simulink model "TorqueCtrl"  (R2022b)
settings: Solver=FixedStepDiscrete  StartTime=0.0  StopTime=10.0  RelTol=1e-3
values from neighbouring files (symbols this model uses):
  C_TorqueCtrl_MaxTrqIndex_u16 = 0.0    [TorqueCtrl.sldd]    (also in TorqueCtrl_objects.m = myPackage.Parameter)
  C_TorqueCtrl_MaxTrqTable_u16 = 0.0    [TorqueCtrl.sldd]    (also in TorqueCtrl_objects.m = myPackage.Parameter)
  C_TorqueCtrl_PowerCoeff60V_u16 = 0.0    [TorqueCtrl.sldd]    (also in TorqueCtrl_objects.m = myPackage.Parameter)
  C_TorqueCtrl_PowerCoeff72V_u16 = 0.0    [TorqueCtrl.sldd]    (also in TorqueCtrl_objects.m = myPackage.Parameter)
undefined symbols (not defined in the file or in its folder): ANALOG, cSpeedLoopMode, cTorqueLoopMode, MOTORDIR, ParamCfg_CommandSource_u16, ParamCfg_MaxSpeed_u16, ParamCfg_PowerMax_u16, ParamCfg_PowerMaxNeg_u16, ParamCfg_Spdouttype_u16, ParamCfg_SpeedKi_u16, ParamCfg_SpeedKp_u16
libraries: simulink x11, YS_UserDefined_Library x1
settings Model: DataDictionary=TorqueCtrl.sldd  Creator=ZYH  LastModifiedBy=ZYH
settings OptimizationCC: DefaultParameterBehavior=Inlined  EnhancedBackFolding=on  PassReuseOutputArgsAs=Individual arguments  ZeroExternalMemoryAtStartup=off  ZeroInternalMemoryAtStartup=off  OptimizeBlockOrder=speed  DifferentSizesBufferReuse=on  OptimizationCustomize=off  EfficientTunableParamExpr=on
settings DebuggingCC: ParameterTunabilityLossMsg=error
settings SFSimCC: MATLABDynamicMemAlloc=off
settings RTWCC: Description=Embedded Coder  SystemTargetFile=ert.tlc  GenCodeOnly=on  TemplateMakefile=ert_default_tmf
settings CodeAppCC: ForceParamTrailComments=on  IgnoreCustomStorageClasses=off  OperatorAnnotations=on  SimulinkDataObjDesc=on  SFDataObjDesc=on  InsertBlockDesc=on
settings ERTTargetCC: TargetLangStandard=C99 (ISO)  GenerateSampleERTMain=on  InlinedParameterPlacement=NonHierarchical  ERTCustomFileTemplate=example_file_process.tlc

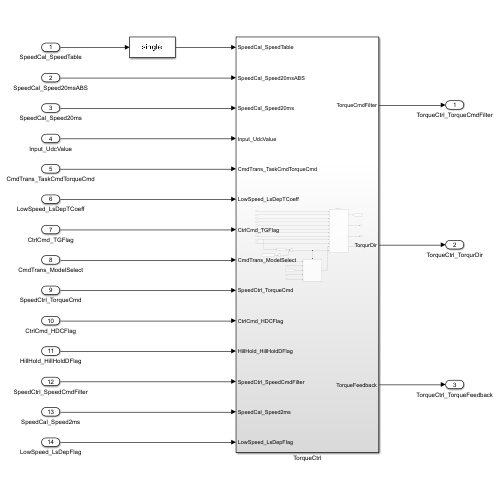
[thumbnail: Simulink's stored preview of the top-level diagram]
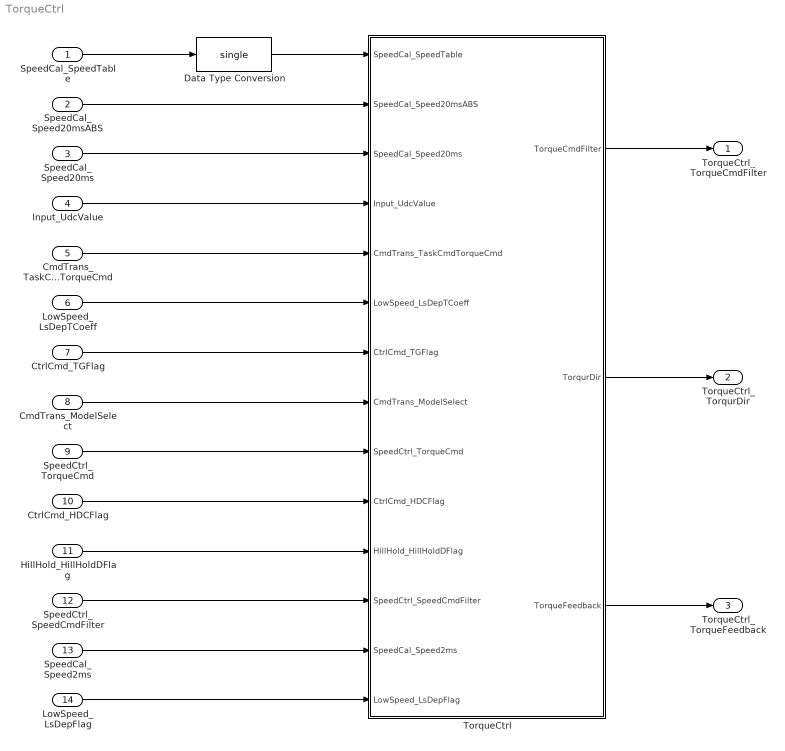
== system TorqueCtrl ==
  SpeedCal_SpeedTable : Inport
  SpeedCal_Speed20msABS : Inport  Port=2
  SpeedCal_Speed20ms : Inport  Port=3
  Input_UdcValue : Inport  Port=4
  CmdTrans_TaskCmdTorqueCmd : Inport  Port=5
  LowSpeed_LsDepTCoeff : Inport  Port=6
  CtrlCmd_TGFlag : Inport  Port=7
  CmdTrans_ModelSelect : Inport  Port=8
  SpeedCtrl_TorqueCmd : Inport  Port=9
  CtrlCmd_HDCFlag : Inport  Port=10
  HillHold_HillHoldDFlag : Inport  Port=11
  SpeedCtrl_SpeedCmdFilter : Inport  Port=12
  SpeedCal_Speed2ms : Inport  Port=13
  LowSpeed_LsDepFlag : Inport  Port=14
  Data Type Conversion : DataTypeConversion  OutDataTypeStr=single  SaturateOnIntegerOverflow=off  RndMeth=Floor
  TorqueCtrl : Subsystem
  TorqueCtrl_TorqueCmdFilter : Outport
  TorqueCtrl_TorqurDir : Outport  Port=2
  TorqueCtrl_TorqueFeedback : Outport  Port=3
  wires:
  SpeedCal_SpeedTable/1 -> Data Type Conversion/1
  Data Type Conversion/1 -> TorqueCtrl/1(SpeedCal_SpeedTable)
  SpeedCal_Speed20msABS/1 -> TorqueCtrl/2(SpeedCal_Speed20msABS)
  Input_UdcValue/1 -> TorqueCtrl/4(Input_UdcValue)
  CmdTrans_TaskCmdTorqueCmd/1 -> TorqueCtrl/5(CmdTrans_TaskCmdTorqueCmd)
  SpeedCal_Speed20ms/1 -> TorqueCtrl/3(SpeedCal_Speed20ms)
  LowSpeed_LsDepTCoeff/1 -> TorqueCtrl/6(LowSpeed_LsDepTCoeff)
  SpeedCtrl_TorqueCmd/1 -> TorqueCtrl/9(SpeedCtrl_TorqueCmd)
  CmdTrans_ModelSelect/1 -> TorqueCtrl/8(CmdTrans_ModelSelect)
  CtrlCmd_TGFlag/1 -> TorqueCtrl/7(CtrlCmd_TGFlag)
  TorqueCtrl/1(TorqueCmdFilter) -> TorqueCtrl_TorqueCmdFilter/1
  TorqueCtrl/2(TorqurDir) -> TorqueCtrl_TorqurDir/1
  TorqueCtrl/3(TorqueFeedback) -> TorqueCtrl_TorqueFeedback/1
  CtrlCmd_HDCFlag/1 -> TorqueCtrl/10(CtrlCmd_HDCFlag)
  HillHold_HillHoldDFlag/1 -> TorqueCtrl/11(HillHold_HillHoldDFlag)
  SpeedCtrl_SpeedCmdFilter/1 -> TorqueCtrl/12(SpeedCtrl_SpeedCmdFilter)
  SpeedCal_Speed2ms/1 -> TorqueCtrl/13(SpeedCal_Speed2ms)
  LowSpeed_LsDepFlag/1 -> TorqueCtrl/14(LowSpeed_LsDepFlag)

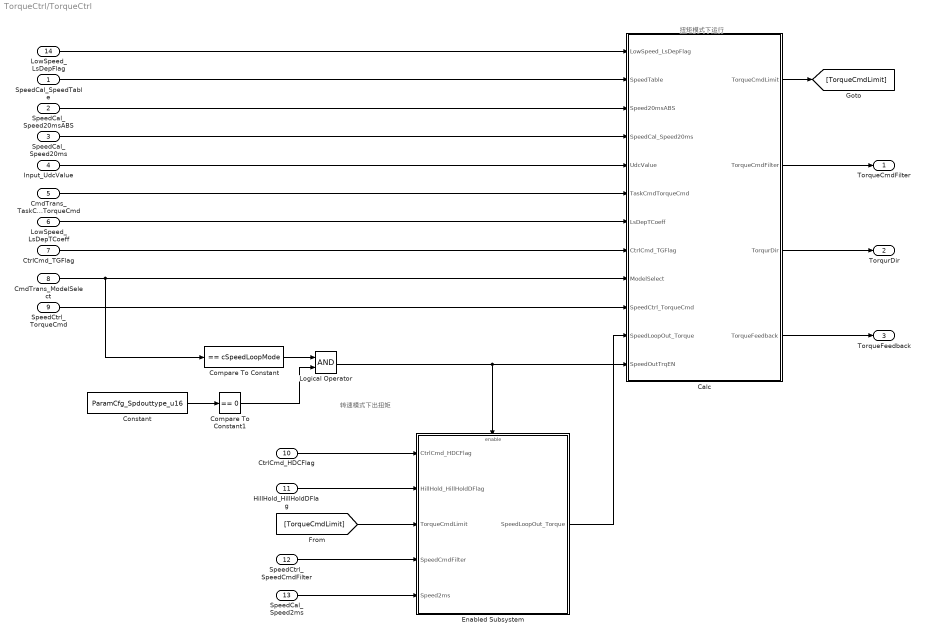
== system TorqueCtrl/TorqueCtrl ==
  note: 转速模式下出扭矩
  note: 扭矩模式下运行
  SpeedCal_SpeedTable : Inport
  SpeedCal_Speed20msABS : Inport  Port=2
  SpeedCal_Speed20ms : Inport  Port=3
  Input_UdcValue : Inport  Port=4
  CmdTrans_TaskCmdTorqueCmd : Inport  Port=5
  LowSpeed_LsDepTCoeff : Inport  Port=6
  CtrlCmd_TGFlag : Inport  Port=7
  CmdTrans_ModelSelect : Inport  Port=8
  SpeedCtrl_TorqueCmd : Inport  Port=9
  CtrlCmd_HDCFlag : Inport  Port=10
  HillHold_HillHoldDFlag : Inport  Port=11
  SpeedCtrl_SpeedCmdFilter : Inport  Port=12
  SpeedCal_Speed2ms : Inport  Port=13
  LowSpeed_LsDepFlag : Inport  Port=14
  Calc : Subsystem
  Compare To Constant : simulink/Logic and Bit Operations/Compare To Constant  relop===  const=cSpeedLoopMode  OutDataTypeStr=boolean
  Compare To Constant1 : simulink/Logic and Bit Operations/Compare To Constant  relop===  const=0  OutDataTypeStr=boolean
  Constant : Constant  Value=ParamCfg_Spdouttype_u16
  Enabled Subsystem : Subsystem  TreatAsAtomicUnit=on
  Logical Operator : Logic  AllPortsSameDT=off  OutDataTypeStr=boolean
  TorqueCmdFilter : Outport
  TorqurDir : Outport  Port=2
  TorqueFeedback : Outport  Port=3
  wires:
  SpeedCal_SpeedTable/1 -> Calc/2(SpeedTable)
  SpeedCal_Speed20msABS/1 -> Calc/3(Speed20msABS)
  Input_UdcValue/1 -> Calc/5(UdcValue)
  CmdTrans_TaskCmdTorqueCmd/1 -> Calc/6(TaskCmdTorqueCmd)
  SpeedCal_Speed20ms/1 -> Calc/4(SpeedCal_Speed20ms)
  LowSpeed_LsDepTCoeff/1 -> Calc/7(LsDepTCoeff)
  CmdTrans_ModelSelect/1 -> Compare To Constant/1, Calc/9(ModelSelect)
  SpeedCtrl_TorqueCmd/1 -> Calc/10(SpeedCtrl_TorqueCmd)
  CtrlCmd_TGFlag/1 -> Calc/8(CtrlCmd_TGFlag)
  Calc/1(TorqueCmdLimit) -> [TorqueCmdLimit]
  Calc/2(TorqueCmdFilter) -> TorqueCmdFilter/1
  Calc/3(TorqurDir) -> TorqurDir/1
  Calc/4(TorqueFeedback) -> TorqueFeedback/1
  Compare To Constant/1 -> Logical Operator/1
  Logical Operator/1 -> Enabled Subsystem/Enable, Calc/12(SpeedOutTrqEN)
  Constant/1 -> Compare To Constant1/1
  Compare To Constant1/1 -> Logical Operator/2
  CtrlCmd_HDCFlag/1 -> Enabled Subsystem/1(CtrlCmd_HDCFlag)
  HillHold_HillHoldDFlag/1 -> Enabled Subsystem/2(HillHold_HillHoldDFlag)
  [TorqueCmdLimit] -> Enabled Subsystem/3(TorqueCmdLimit)
  SpeedCtrl_SpeedCmdFilter/1 -> Enabled Subsystem/4(SpeedCmdFilter)
  SpeedCal_Speed2ms/1 -> Enabled Subsystem/5(Speed2ms)
  Enabled Subsystem/1(SpeedLoopOut_Torque) -> Calc/11(SpeedLoopOut_Torque)
  LowSpeed_LsDepFlag/1 -> Calc/1(LowSpeed_LsDepFlag)

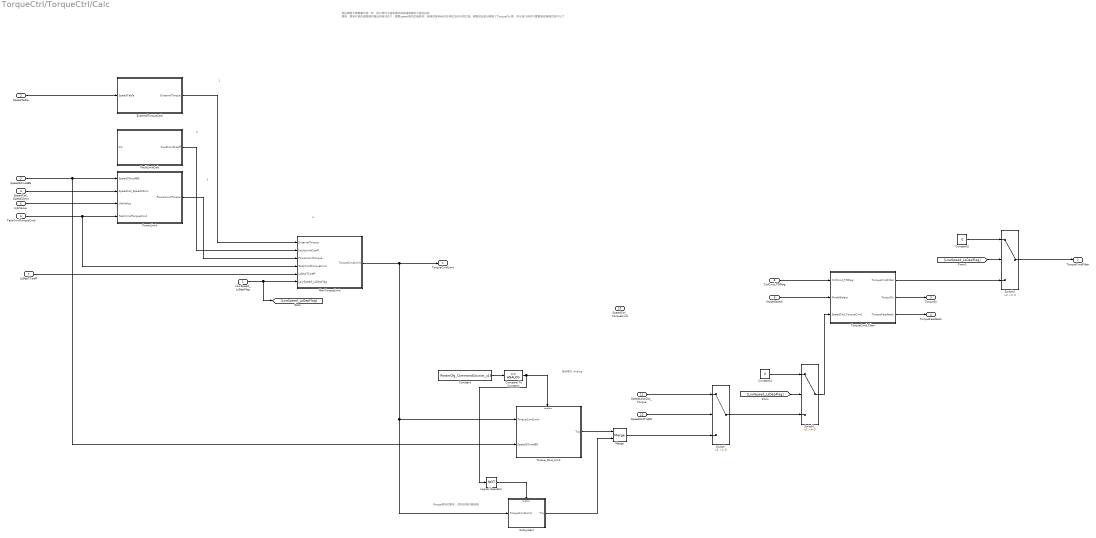
== system TorqueCtrl/TorqueCtrl/Calc ==
  note: 现在模型不需要像代码一样，执行条件为扭矩模式或者速度模式下输出扭矩
      |
      | 原因：原来代码在速度模式输出扭矩状态下，需要speed相关的函数判断是否是ANALOG模式去执行防打滑。模型把这部分挪到了TorqueCtrl里，所以执行条件只需要是扭矩模式就可以了
  note: 4
  note: 3
  note: 2
  note: 1
  note: Merge模块的要求，否则仿真时候报错
  note: 扭矩模式
      | 	Analog
  LowSpeed_LsDepFlag : Inport
  SpeedTable : Inport  Port=2
  Speed20msABS : Inport  Port=3
  SpeedCal_Speed20ms : Inport  Port=4
  UdcValue : Inport  Port=5
  TaskCmdTorqueCmd : Inport  Port=6
  LsDepTCoeff : Inport  Port=7
  CtrlCmd_TGFlag : Inport  Port=8
  ModelSelect : Inport  Port=9
  SpeedCtrl_TorqueCmd : Inport  Port=10
  SpeedLoopOut_Torque : Inport  Port=11
  SpeedOutTrqEN : Inport  Port=12
  Compare To Constant : simulink/Logic and Bit Operations/Compare To Constant  relop===  const=ANALOG  OutDataTypeStr=boolean
  Constant : Constant  Value=ParamCfg_CommandSource_u16
  Constant1 : Constant  Value=0  OutDataTypeStr=single
  Constant2 : Constant  Value=0  OutDataTypeStr=single
  ExternalTorqueCalc : Subsystem
  FaultLimitCalc : Subsystem
  Logical Operator : Logic  Operator=NOT  AllPortsSameDT=off  OutDataTypeStr=boolean
  MaxTorqueLimit : Subsystem
  Merge : Merge
  PowerLimit : Subsystem
  Subsystem : Subsystem
  Switch : Switch  Criteria=u2 ~= 0  SaturateOnIntegerOverflow=off  InputSameDT=off
  Switch1 : Switch  Criteria=u2 ~= 0  SaturateOnIntegerOverflow=off  InputSameDT=off
  Switch2 : Switch  Criteria=u2 ~= 0  SaturateOnIntegerOverflow=off  InputSameDT=off
  TorqueCmd_Filter : Subsystem
  Torque_Skid_Limit : Subsystem
  TorqueCmdLimit : Outport
  TorqueCmdFilter : Outport  Port=2
  TorqurDir : Outport  Port=3
  TorqueFeedback : Outport  Port=4
  wires:
  SpeedTable/1 -> ExternalTorqueCalc/1(SpeedTable)
  Speed20msABS/1 -> Torque_Skid_Limit/2(Speed20msABS), PowerLimit/1(Speed20msABS)
  UdcValue/1 -> PowerLimit/3(UdcValue)
  TaskCmdTorqueCmd/1 -> MaxTorqueLimit/4(TaskCmdTorqueCmd), PowerLimit/4(TaskCmdTorqueCmd)
  SpeedCal_Speed20ms/1 -> PowerLimit/2(SpeedCal_Speed20ms)
  LsDepTCoeff/1 -> MaxTorqueLimit/5(LsDepTCoeff)
  FaultLimitCalc/1(FaultLimitCoeff) -> MaxTorqueLimit/2(FaultLimitCoeff)
  ExternalTorqueCalc/1(ExternalTorque) -> MaxTorqueLimit/1(ExternalTorque)
  PowerLimit/1(PowerLimitTorque) -> MaxTorqueLimit/3(PowerLimitTorque)
  CtrlCmd_TGFlag/1 -> TorqueCmd_Filter/1(CtrlCmd_TGFlag)
  ModelSelect/1 -> TorqueCmd_Filter/2(ModelSelect)
  Switch2/1 -> TorqueCmdFilter/1
  TorqueCmd_Filter/2(TorqurDir) -> TorqurDir/1
  TorqueCmd_Filter/3(TorqueFeedback) -> TorqueFeedback/1
  MaxTorqueLimit/1(TorqueCmdLimit) -> Torque_Skid_Limit/1(TorqueCmdLimit), Subsystem/1(TorqueCmdLimit), TorqueCmdLimit/1
  Constant/1 -> Compare To Constant/1
  Torque_Skid_Limit/1(Trq) -> Merge/1
  Subsystem/1(Trq) -> Merge/2
  Compare To Constant/1 -> Logical Operator/1, Torque_Skid_Limit/Enable
  Logical Operator/1 -> Subsystem/Enable
  Switch/1 -> Switch1/3
  SpeedLoopOut_Torque/1 -> Switch/1
  Merge/1 -> Switch/3
  SpeedOutTrqEN/1 -> Switch/2
  LowSpeed_LsDepFlag/1 -> [LowSpeed_LsDepFlag], MaxTorqueLimit/6(LowSpeed_LsDepFlag)
  [LowSpeed_LsDepFlag] -> Switch1/2
  Constant1/1 -> Switch1/1
  Switch1/1 -> TorqueCmd_Filter/3(SpeedCtrl_TorqueCmd)
  TorqueCmd_Filter/1(TorqueCmdFilter) -> Switch2/3
  [LowSpeed_LsDepFlag] -> Switch2/2
  Constant2/1 -> Switch2/1

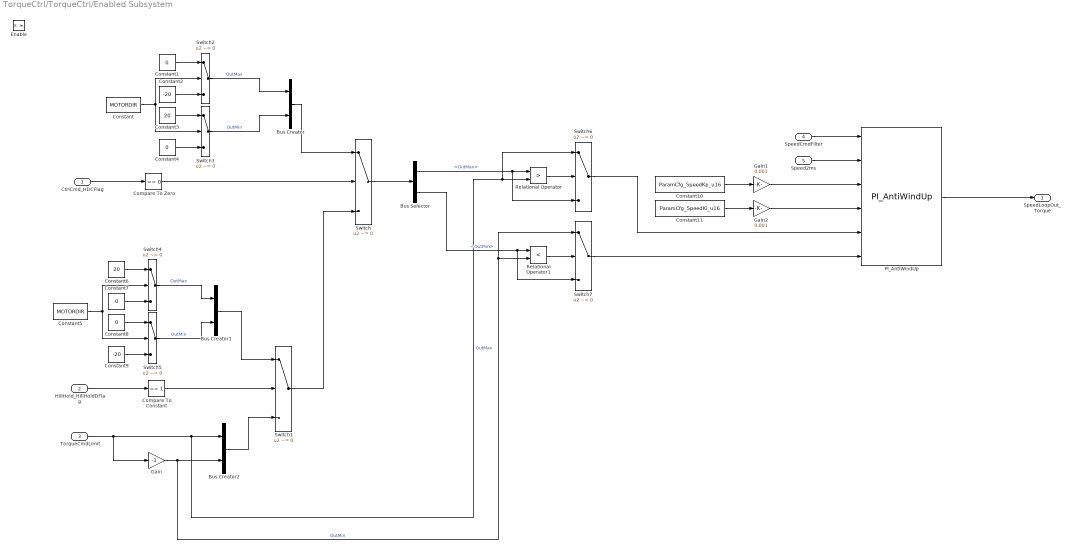
== system TorqueCtrl/TorqueCtrl/Enabled Subsystem ==
  CtrlCmd_HDCFlag : Inport
  HillHold_HillHoldDFlag : Inport  Port=2
  TorqueCmdLimit : Inport  Port=3
  SpeedCmdFilter : Inport  Port=4
  Speed2ms : Inport  Port=5
  Enable : EnablePort
  Bus Creator : BusCreator  Inputs=2
  Bus Creator1 : BusCreator  Inputs=2
  Bus Creator2 : BusCreator  Inputs=2
  Bus Selector : BusSelector  OutputSignals=OutMax,OutMin
  Compare To Constant : simulink/Logic and Bit Operations/Compare To Constant  relop===  const=1  OutDataTypeStr=boolean
  Compare To Zero : simulink/Logic and Bit Operations/Compare To Zero  relop===  OutDataTypeStr=boolean
  Constant : Constant  Value=MOTORDIR
  Constant{1,4,7..8} (4 alike) : Constant  Value=0  OutDataTypeStr=single
  Constant10 : Constant  Value=ParamCfg_SpeedKp_u16
  Constant11 : Constant  Value=ParamCfg_SpeedKi_u16
  Constant2 : Constant  Value=-20  OutDataTypeStr=single
  Constant3 : Constant  Value=20  OutDataTypeStr=single
  Constant5 : Constant  Value=MOTORDIR
  Constant6 : Constant  Value=20  OutDataTypeStr=single
  Constant9 : Constant  Value=-20  OutDataTypeStr=single
  Gain : Gain  Gain=-1  ParamDataTypeStr=single  OutDataTypeStr=single
  Gain1 : Gain  Gain=0.001  ParamDataTypeStr=single  OutDataTypeStr=single
      settings: AttributesFormatString=%<Gain>
  Gain2 : Gain  Gain=0.001  ParamDataTypeStr=single  OutDataTypeStr=single
      settings: AttributesFormatString=%<Gain>
  PI_AntiWindUp : YS_UserDefined_Library/PID/PI_AntiWindUp
      settings: SourceProductName=YS
  Relational Operator : RelationalOperator  Operator=>  OutDataTypeStr=boolean  RndMeth=Simplest  InputSameDT=off
  Relational Operator1 : RelationalOperator  Operator=<  OutDataTypeStr=boolean  RndMeth=Simplest  InputSameDT=off
  Switch{,1..7} (8 alike) : Switch  Criteria=u2 ~= 0  SaturateOnIntegerOverflow=off  InputSameDT=off
  SpeedLoopOut_Torque : Outport
  wires:
  CtrlCmd_HDCFlag/1 -> Compare To Zero/1
  Compare To Zero/1 -> Switch/2
  Bus Creator/1 -> Switch/1
  HillHold_HillHoldDFlag/1 -> Compare To Constant/1
  Compare To Constant/1 -> Switch1/2
  Switch1/1 -> Switch/3
  Constant1/1 -> Switch2/1
  Constant2/1 -> Switch2/3
  Constant3/1 -> Switch3/1
  Constant4/1 -> Switch3/3
  Switch2/1 -> Bus Creator/1  "OutMax"
  Switch3/1 -> Bus Creator/2  "OutMin"
  Constant/1 -> Switch2/2, Switch3/2
  Switch5/1 -> Bus Creator1/2  "OutMin"
  Switch4/1 -> Bus Creator1/1  "OutMax"
  Constant8/1 -> Switch5/1
  Constant5/1 -> Switch4/2, Switch5/2
  Constant9/1 -> Switch5/3
  Constant6/1 -> Switch4/1
  Constant7/1 -> Switch4/3
  Bus Creator1/1 -> Switch1/1
  Bus Creator2/1 -> Switch1/3
  TorqueCmdLimit/1 -> Gain/1, Switch6/1, Relational Operator/2, Bus Creator2/1  "OutMax"
  Gain/1 -> Switch7/1, Relational Operator1/2, Bus Creator2/2  "OutMin"
  Switch/1 -> Bus Selector/1
  Bus Selector/1 -> Switch6/3, Relational Operator/1  "<OutMax>"
  Bus Selector/2 -> Switch7/3, Relational Operator1/1  "<OutMin>"
  Relational Operator/1 -> Switch6/2
  Relational Operator1/1 -> Switch7/2
  Switch6/1 -> PI_AntiWindUp/5
  PI_AntiWindUp/1 -> SpeedLoopOut_Torque/1
  Switch7/1 -> PI_AntiWindUp/6
  SpeedCmdFilter/1 -> PI_AntiWindUp/1
  Speed2ms/1 -> PI_AntiWindUp/2
  Constant10/1 -> Gain1/1
  Gain1/1 -> PI_AntiWindUp/3
  Gain2/1 -> PI_AntiWindUp/4
  Constant11/1 -> Gain2/1

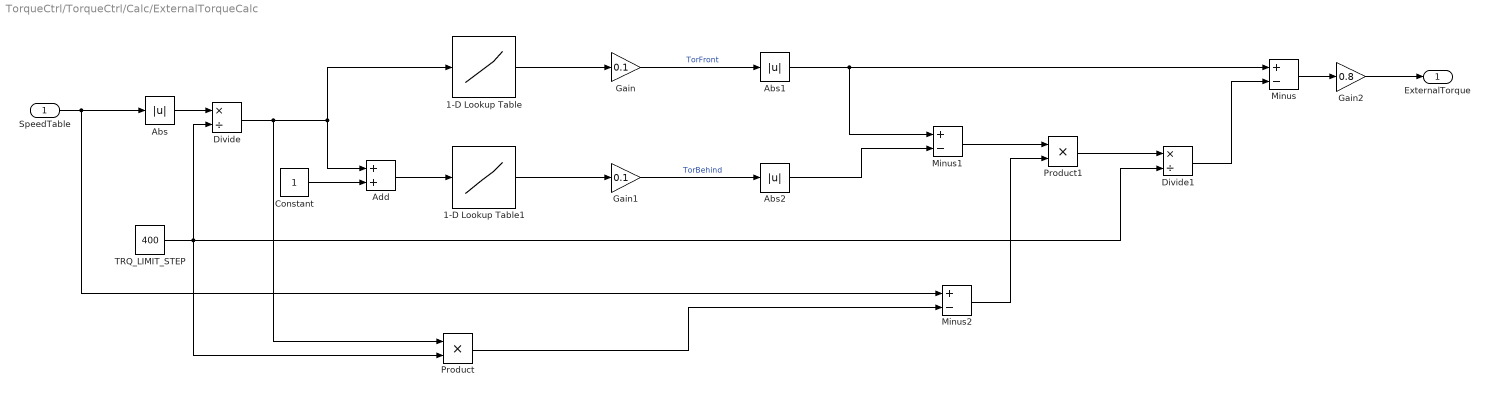
== system TorqueCtrl/TorqueCtrl/Calc/ExternalTorqueCalc ==
  SpeedTable : Inport
  1-D Lookup Table : Lookup_n-D  NumberOfTableDimensions=1  BreakpointsForDimension1=C_TorqueCtrl_MaxTrqIndex_u16  BreakpointsForDimension1DataTypeStr=Inherit: Inherit from 'Breakpoint data'  Table=C_TorqueCtrl_MaxTrqTable_u16  TableDataTypeStr=Inherit: Inherit from 'Table data'  ExtrapMethod=Clip  InternalRulePriority=Speed  OutDataTypeStr=Inherit: Inherit from 'Table data'  RndMeth=Simplest
  1-D Lookup Table1 : Lookup_n-D  NumberOfTableDimensions=1  BreakpointsForDimension1=C_TorqueCtrl_MaxTrqIndex_u16  BreakpointsForDimension1DataTypeStr=Inherit: Inherit from 'Breakpoint data'  Table=C_TorqueCtrl_MaxTrqTable_u16  TableDataTypeStr=Inherit: Inherit from 'Table data'  ExtrapMethod=Clip  InternalRulePriority=Speed  OutDataTypeStr=Inherit: Inherit from 'Table data'  RndMeth=Simplest
  Abs : Abs  SaturateOnIntegerOverflow=off
  Abs1 : Abs  SaturateOnIntegerOverflow=off
  Abs2 : Abs  SaturateOnIntegerOverflow=off
  Add : Sum
  Constant : Constant  OutDataTypeStr=uint16
  Divide : Product  Inputs=*/  OutDataTypeStr=uint16
  Divide1 : Product  Inputs=*/
  Gain : Gain  Gain=0.1  ParamDataTypeStr=single  OutDataTypeStr=single
  Gain1 : Gain  Gain=0.1  ParamDataTypeStr=single  OutDataTypeStr=single
  Gain2 : Gain  Gain=0.8  ParamDataTypeStr=single  OutDataTypeStr=single
  Minus : Sum  Inputs=+-
  Minus1 : Sum  Inputs=+-
  Minus2 : Sum  Inputs=+-
  Product : Product
  Product1 : Product
  TRQ_LIMIT_STEP : Constant  Value=400  OutDataTypeStr=uint16
  ExternalTorque : Outport
  wires:
  TRQ_LIMIT_STEP/1 -> Divide1/2, Divide/2, Product/2
  SpeedTable/1 -> Minus2/1, Abs/1
  Abs/1 -> Divide/1
  Divide/1 -> Product/1, Add/1, 1-D Lookup Table/1
  Constant/1 -> Add/2
  Add/1 -> 1-D Lookup Table1/1
  1-D Lookup Table/1 -> Gain/1
  Gain/1 -> Abs1/1  "TorFront"
  1-D Lookup Table1/1 -> Gain1/1
  Gain1/1 -> Abs2/1  "TorBehind"
  Abs1/1 -> Minus1/1, Minus/1
  Abs2/1 -> Minus1/2
  Product/1 -> Minus2/2
  Minus1/1 -> Product1/1
  Minus2/1 -> Product1/2
  Product1/1 -> Divide1/1
  Divide1/1 -> Minus/2
  Minus/1 -> Gain2/1
  Gain2/1 -> ExternalTorque/1

== system TorqueCtrl/TorqueCtrl/Calc/FaultLimitCalc ==
  In1 : Inport
  FaultLimitCoeff : Outport
  wires:
  In1/1 -> FaultLimitCoeff/1

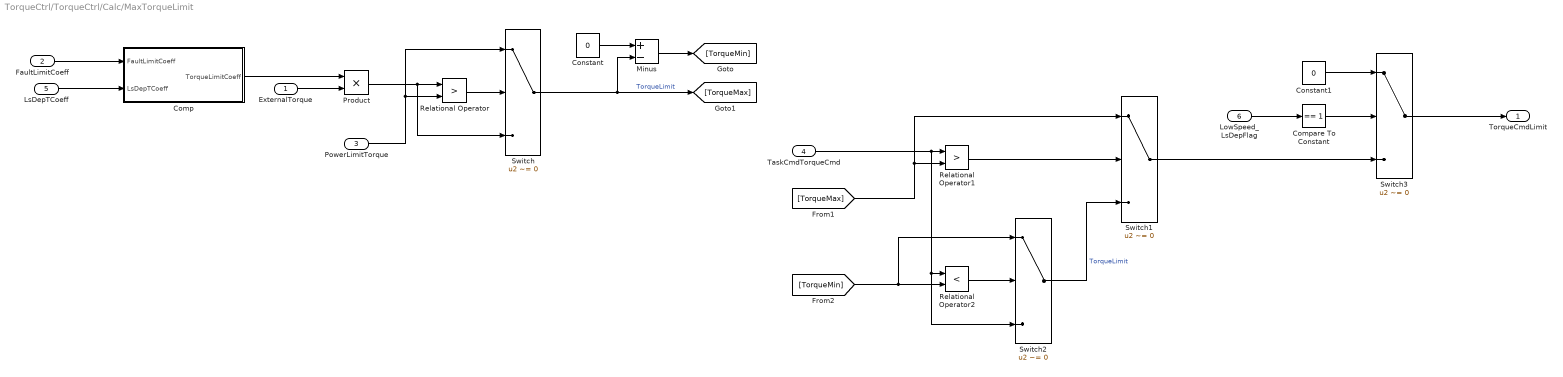
== system TorqueCtrl/TorqueCtrl/Calc/MaxTorqueLimit ==
  ExternalTorque : Inport
  FaultLimitCoeff : Inport  Port=2
  PowerLimitTorque : Inport  Port=3
  TaskCmdTorqueCmd : Inport  Port=4
  LsDepTCoeff : Inport  Port=5
  LowSpeed_LsDepFlag : Inport  Port=6
  Comp : Subsystem
  Compare To Constant : simulink/Logic and Bit Operations/Compare To Constant  relop===  const=1  OutDataTypeStr=boolean
  Constant : Constant  Value=0  OutDataTypeStr=single
  Constant1 : Constant  Value=0  OutDataTypeStr=single
  Minus : Sum  Inputs=+-
  Product : Product  OutDataTypeStr=single
  Relational Operator : RelationalOperator  Operator=>  OutDataTypeStr=boolean  RndMeth=Simplest  InputSameDT=off
  Relational Operator1 : RelationalOperator  Operator=>  OutDataTypeStr=boolean  RndMeth=Simplest  InputSameDT=off
  Relational Operator2 : RelationalOperator  Operator=<  OutDataTypeStr=boolean  RndMeth=Simplest  InputSameDT=off
  Switch{,1..3} (4 alike) : Switch  Criteria=u2 ~= 0  SaturateOnIntegerOverflow=off  InputSameDT=off
  TorqueCmdLimit : Outport
  wires:
  FaultLimitCoeff/1 -> Comp/1(FaultLimitCoeff)
  LsDepTCoeff/1 -> Comp/2(LsDepTCoeff)
  Comp/1(TorqueLimitCoeff) -> Product/1
  ExternalTorque/1 -> Product/2
  Product/1 -> Switch/3, Relational Operator/1
  PowerLimitTorque/1 -> Switch/1, Relational Operator/2
  Relational Operator/1 -> Switch/2
  Switch/1 -> [TorqueMax], Minus/2  "TorqueLimit"
  Constant/1 -> Minus/1
  Minus/1 -> [TorqueMin]
  TaskCmdTorqueCmd/1 -> Switch2/3, Relational Operator2/1, Relational Operator1/1
  [TorqueMax] -> Relational Operator1/2, Switch1/1
  Relational Operator1/1 -> Switch1/2
  [TorqueMin] -> Switch2/1, Relational Operator2/2
  Relational Operator2/1 -> Switch2/2
  Switch2/1 -> Switch1/3  "TorqueLimit"
  Switch1/1 -> Switch3/3
  LowSpeed_LsDepFlag/1 -> Compare To Constant/1
  Compare To Constant/1 -> Switch3/2
  Switch3/1 -> TorqueCmdLimit/1
  Constant1/1 -> Switch3/1

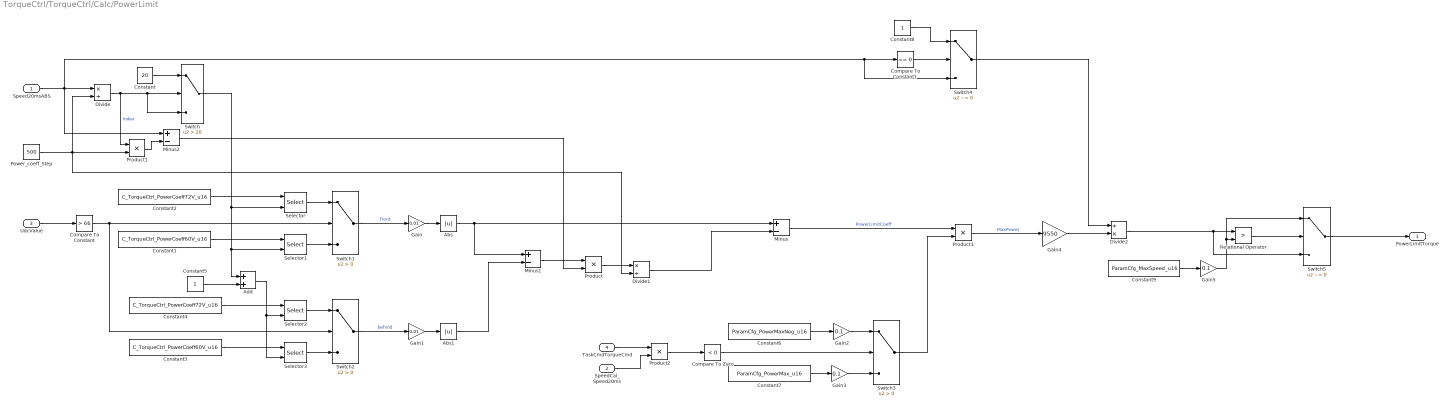
== system TorqueCtrl/TorqueCtrl/Calc/PowerLimit ==
  Speed20msABS : Inport
  SpeedCal_Speed20ms : Inport  Port=2
  UdcValue : Inport  Port=3
  TaskCmdTorqueCmd : Inport  Port=4
  Abs : Abs  SaturateOnIntegerOverflow=off
  Abs1 : Abs  SaturateOnIntegerOverflow=off
  Add : Sum
  Compare To Constant : simulink/Logic and Bit Operations/Compare To Constant  relop=>  const=66  OutDataTypeStr=boolean
  Compare To Constant1 : simulink/Logic and Bit Operations/Compare To Constant  relop===  const=0  OutDataTypeStr=boolean
  Compare To Zero : simulink/Logic and Bit Operations/Compare To Zero  relop=<  OutDataTypeStr=boolean
  Constant : Constant  Value=20  OutDataTypeStr=uint16
  Constant1 : Constant  Value=C_TorqueCtrl_PowerCoeff60V_u16
  Constant2 : Constant  Value=C_TorqueCtrl_PowerCoeff72V_u16
  Constant3 : Constant  Value=C_TorqueCtrl_PowerCoeff60V_u16
  Constant4 : Constant  Value=C_TorqueCtrl_PowerCoeff72V_u16
  Constant5 : Constant  OutDataTypeStr=uint16
  Constant6 : Constant  Value=ParamCfg_PowerMaxNeg_u16
  Constant7 : Constant  Value=ParamCfg_PowerMax_u16
  Constant8 : Constant  OutDataTypeStr=single
  Constant9 : Constant  Value=ParamCfg_MaxSpeed_u16
  Divide : Product  Inputs=*/  OutDataTypeStr=uint16
  Divide1 : Product  Inputs=*/
  Divide2 : Product  Inputs=/*
  Gain : Gain  Gain=0.01  ParamDataTypeStr=single  OutDataTypeStr=single
  Gain1 : Gain  Gain=0.01  ParamDataTypeStr=single  OutDataTypeStr=single
  Gain2 : Gain  Gain=0.1  ParamDataTypeStr=single  OutDataTypeStr=single
  Gain3 : Gain  Gain=0.1  ParamDataTypeStr=single  OutDataTypeStr=single
  Gain4 : Gain  Gain=9550  ParamDataTypeStr=single  OutDataTypeStr=single
  Gain5 : Gain  Gain=0.1  ParamDataTypeStr=single  OutDataTypeStr=single
  Minus : Sum  Inputs=+-
  Minus1 : Sum  Inputs=+-
  Minus2 : Sum  Inputs=+-
  Power_coeff_Step : Constant  Value=500  OutDataTypeStr=uint16
  Product : Product
  Product1 : Product  OutDataTypeStr=uint16
  Product2 : Product
  Product3 : Product
  Relational Operator : RelationalOperator  Operator=>  OutDataTypeStr=boolean  RndMeth=Simplest  InputSameDT=off
  Selector{,1..3} (4 alike) : Selector  IndexMode=Zero-based  InputPortWidth=22  IndexOptions=Starting index (port)  Indices=[1 3]  OutputSizes=1
  Switch : Switch  Criteria=u2 > Threshold  Threshold=20  SaturateOnIntegerOverflow=off  InputSameDT=off
  Switch1 : Switch  Criteria=u2 > Threshold  SaturateOnIntegerOverflow=off  InputSameDT=off
  Switch2 : Switch  Criteria=u2 > Threshold  SaturateOnIntegerOverflow=off  InputSameDT=off
  Switch3 : Switch  Criteria=u2 > Threshold  SaturateOnIntegerOverflow=off  InputSameDT=off
  Switch4 : Switch  Criteria=u2 ~= 0  SaturateOnIntegerOverflow=off  InputSameDT=off
  Switch5 : Switch  Criteria=u2 ~= 0  SaturateOnIntegerOverflow=off  InputSameDT=off
  PowerLimitTorque : Outport
  wires:
  Power_coeff_Step/1 -> Divide1/2, Divide/2, Product1/2
  Divide/1 -> Product1/1, Switch/3, Switch/2  "Index"
  Constant/1 -> Switch/1
  UdcValue/1 -> Compare To Constant/1
  Compare To Constant/1 -> Switch1/2, Switch2/2
  Switch1/1 -> Gain/1  "front"
  Switch2/1 -> Gain1/1  "behind"
  Constant2/1 -> Selector/1
  Switch/1 -> Add/1, Selector1/2, Selector/2
  Selector/1 -> Switch1/1
  Selector1/1 -> Switch1/3
  Constant1/1 -> Selector1/1
  Selector2/1 -> Switch2/1
  Constant5/1 -> Add/2
  Add/1 -> Selector3/2, Selector2/2
  Constant4/1 -> Selector2/1
  Selector3/1 -> Switch2/3
  Constant3/1 -> Selector3/1
  Abs/1 -> Minus1/1, Minus/1
  Abs1/1 -> Minus1/2
  Minus1/1 -> Product/1
  Product1/1 -> Minus2/2
  Minus2/1 -> Product/2
  Product/1 -> Divide1/1
  Gain/1 -> Abs/1
  Gain1/1 -> Abs1/1
  Divide1/1 -> Minus/2
  Minus/1 -> Product3/1  "PowerLimitCoeff"
  TaskCmdTorqueCmd/1 -> Product2/1
  Speed20msABS/1 -> Minus2/1, Switch4/3, Compare To Constant1/1, Divide/1
  SpeedCal_Speed20ms/1 -> Product2/2
  Product2/1 -> Compare To Zero/1
  Compare To Zero/1 -> Switch3/2
  Constant6/1 -> Gain2/1
  Gain2/1 -> Switch3/1
  Constant7/1 -> Gain3/1
  Gain3/1 -> Switch3/3
  Switch3/1 -> Product3/2
  Product3/1 -> Gain4/1  "MaxPower"
  Compare To Constant1/1 -> Switch4/2
  Constant8/1 -> Switch4/1
  Gain4/1 -> Divide2/2
  Switch4/1 -> Divide2/1
  Constant9/1 -> Gain5/1
  Divide2/1 -> Switch5/3, Relational Operator/1
  Gain5/1 -> Switch5/1, Relational Operator/2
  Relational Operator/1 -> Switch5/2
  Switch5/1 -> PowerLimitTorque/1

== system TorqueCtrl/TorqueCtrl/Calc/Subsystem ==
  TorqueCmdLimit : Inport
  Enable : EnablePort
  Trq : Outport
  wires:
  TorqueCmdLimit/1 -> Trq/1

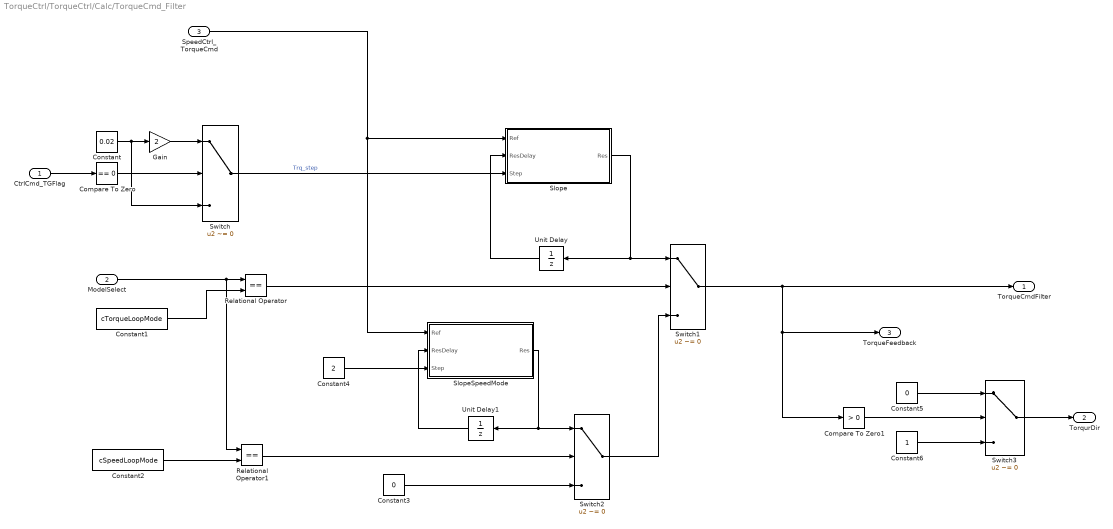
== system TorqueCtrl/TorqueCtrl/Calc/TorqueCmd_Filter ==
  CtrlCmd_TGFlag : Inport
  ModelSelect : Inport  Port=2
  SpeedCtrl_TorqueCmd : Inport  Port=3
  Compare To Zero : simulink/Logic and Bit Operations/Compare To Zero  relop===  OutDataTypeStr=boolean
  Compare To Zero1 : simulink/Logic and Bit Operations/Compare To Zero  relop=>  OutDataTypeStr=boolean
  Constant : Constant  Value=0.02  OutDataTypeStr=single
  Constant1 : Constant  Value=cTorqueLoopMode
  Constant2 : Constant  Value=cSpeedLoopMode
  Constant3 : Constant  Value=0  OutDataTypeStr=single
  Constant4 : Constant  Value=2  OutDataTypeStr=single
  Constant5 : Constant  Value=0  OutDataTypeStr=uint8
  Constant6 : Constant  OutDataTypeStr=uint8
  Gain : Gain  Gain=2  ParamDataTypeStr=single  OutDataTypeStr=single
  Relational Operator : RelationalOperator  Operator===  OutDataTypeStr=boolean  RndMeth=Simplest  InputSameDT=off
  Relational Operator1 : RelationalOperator  Operator===  OutDataTypeStr=boolean  RndMeth=Simplest  InputSameDT=off
  Slope : Subsystem
  SlopeSpeedMode : Subsystem
  Switch{,1..3} (4 alike) : Switch  Criteria=u2 ~= 0  SaturateOnIntegerOverflow=off  InputSameDT=off
  Unit Delay : UnitDelay  SampleTime=-1  HasFrameUpgradeWarning=on
  Unit Delay1 : UnitDelay  SampleTime=-1  HasFrameUpgradeWarning=on
  TorqueCmdFilter : Outport
  TorqurDir : Outport  Port=2
  TorqueFeedback : Outport  Port=3
  wires:
  CtrlCmd_TGFlag/1 -> Compare To Zero/1
  Compare To Zero/1 -> Switch/2
  Constant/1 -> Switch/3, Gain/1
  Gain/1 -> Switch/1
  Switch/1 -> Slope/3(Step)  "Trq_step"
  ModelSelect/1 -> Relational Operator1/1, Relational Operator/1
  Constant1/1 -> Relational Operator/2
  Relational Operator/1 -> Switch1/2
  SpeedCtrl_TorqueCmd/1 -> Slope/1(Ref), SlopeSpeedMode/1(Ref)
  Slope/1(Res) -> Switch1/1, Unit Delay/1
  Unit Delay/1 -> Slope/2(ResDelay)
  Constant2/1 -> Relational Operator1/2
  Relational Operator1/1 -> Switch2/2
  Switch2/1 -> Switch1/3
  Constant3/1 -> Switch2/3
  SlopeSpeedMode/1(Res) -> Unit Delay1/1, Switch2/1
  Unit Delay1/1 -> SlopeSpeedMode/2(ResDelay)
  Constant4/1 -> SlopeSpeedMode/3(Step)
  Switch1/1 -> TorqueFeedback/1, Compare To Zero1/1, TorqueCmdFilter/1
  Compare To Zero1/1 -> Switch3/2
  Constant5/1 -> Switch3/1
  Constant6/1 -> Switch3/3
  Switch3/1 -> TorqurDir/1

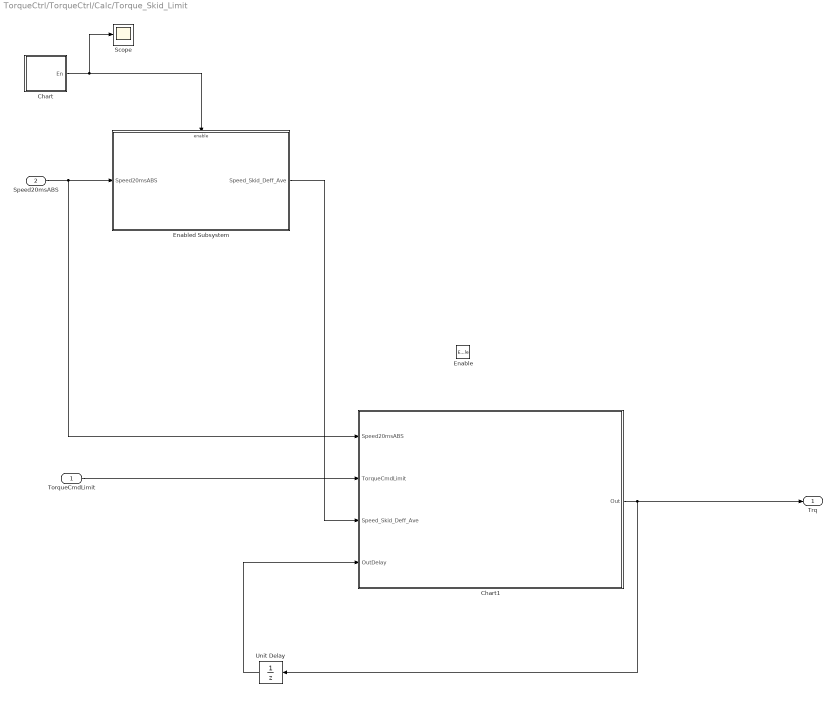
== system TorqueCtrl/TorqueCtrl/Calc/Torque_Skid_Limit ==
  TorqueCmdLimit : Inport
  Speed20msABS : Inport  Port=2
  Enable : EnablePort
  Chart : Stateflow chart  TreatAsAtomicUnit=on
  Chart1 : Stateflow chart  TreatAsAtomicUnit=on
  Enabled Subsystem : Subsystem  TreatAsAtomicUnit=on
  Scope : Scope
  Unit Delay : UnitDelay  SampleTime=-1  HasFrameUpgradeWarning=on
  Trq : Outport
  wires:
  Chart/1(En) -> Scope/1, Enabled Subsystem/Enable
  Speed20msABS/1 -> Chart1/1(Speed20msABS), Enabled Subsystem/1(Speed20msABS)
  TorqueCmdLimit/1 -> Chart1/2(TorqueCmdLimit)
  Chart1/1(Out) -> Trq/1, Unit Delay/1
  Unit Delay/1 -> Chart1/4(OutDelay)
  Enabled Subsystem/1(Speed_Skid_Deff_Ave) -> Chart1/3(Speed_Skid_Deff_Ave)

== system TorqueCtrl/TorqueCtrl/Calc/MaxTorqueLimit/Comp ==
  FaultLimitCoeff : Inport
  LsDepTCoeff : Inport  Port=2
  Relational Operator : RelationalOperator  Operator=<  OutDataTypeStr=boolean  RndMeth=Simplest  InputSameDT=off
  Switch : Switch  Criteria=u2 ~= 0  SaturateOnIntegerOverflow=off  InputSameDT=off
  TorqueLimitCoeff : Outport
  wires:
  LsDepTCoeff/1 -> Switch/1, Relational Operator/1
  FaultLimitCoeff/1 -> Switch/3, Relational Operator/2
  Relational Operator/1 -> Switch/2
  Switch/1 -> TorqueLimitCoeff/1

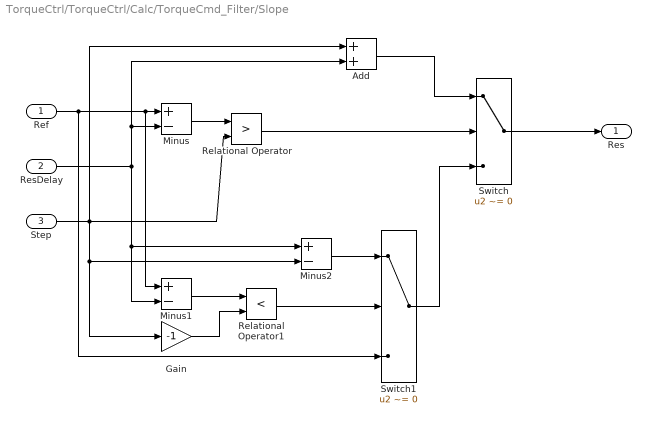
== system TorqueCtrl/TorqueCtrl/Calc/TorqueCmd_Filter/Slope ==
  Ref : Inport
  ResDelay : Inport  Port=2
  Step : Inport  Port=3
  Add : Sum
  Gain : Gain  Gain=-1  ParamDataTypeStr=single  OutDataTypeStr=single
  Minus : Sum  Inputs=+-
  Minus1 : Sum  Inputs=+-
  Minus2 : Sum  Inputs=+-
  Relational Operator : RelationalOperator  Operator=>  OutDataTypeStr=boolean  RndMeth=Simplest  InputSameDT=off
  Relational Operator1 : RelationalOperator  Operator=<  OutDataTypeStr=boolean  RndMeth=Simplest  InputSameDT=off
  Switch : Switch  Criteria=u2 ~= 0  SaturateOnIntegerOverflow=off  InputSameDT=off
  Switch1 : Switch  Criteria=u2 ~= 0  SaturateOnIntegerOverflow=off  InputSameDT=off
  Res : Outport
  wires:
  Ref/1 -> Switch1/3, Minus1/1, Minus/1
  ResDelay/1 -> Minus1/2, Minus2/1, Add/2, Minus/2
  Step/1 -> Minus2/2, Gain/1, Add/1, Relational Operator/2
  Minus/1 -> Relational Operator/1
  Relational Operator/1 -> Switch/2
  Add/1 -> Switch/1
  Minus1/1 -> Relational Operator1/1
  Gain/1 -> Relational Operator1/2
  Relational Operator1/1 -> Switch1/2
  Minus2/1 -> Switch1/1
  Switch1/1 -> Switch/3
  Switch/1 -> Res/1

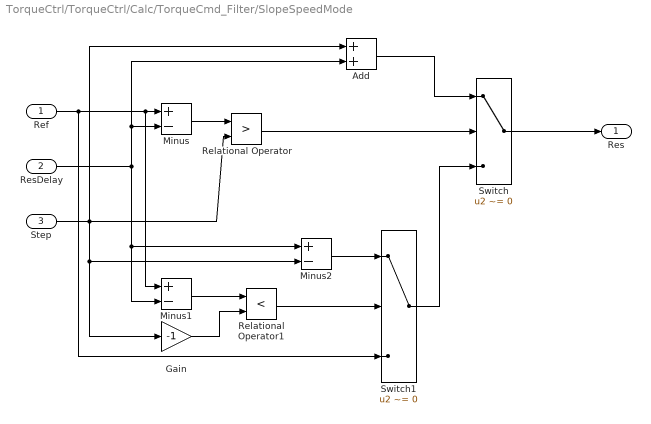
== system TorqueCtrl/TorqueCtrl/Calc/TorqueCmd_Filter/SlopeSpeedMode ==
  Ref : Inport
  ResDelay : Inport  Port=2
  Step : Inport  Port=3
  Add : Sum
  Gain : Gain  Gain=-1  ParamDataTypeStr=single  OutDataTypeStr=single
  Minus : Sum  Inputs=+-
  Minus1 : Sum  Inputs=+-
  Minus2 : Sum  Inputs=+-
  Relational Operator : RelationalOperator  Operator=>  OutDataTypeStr=boolean  RndMeth=Simplest  InputSameDT=off
  Relational Operator1 : RelationalOperator  Operator=<  OutDataTypeStr=boolean  RndMeth=Simplest  InputSameDT=off
  Switch : Switch  Criteria=u2 ~= 0  SaturateOnIntegerOverflow=off  InputSameDT=off
  Switch1 : Switch  Criteria=u2 ~= 0  SaturateOnIntegerOverflow=off  InputSameDT=off
  Res : Outport
  wires:
  Switch/1 -> Res/1
  Switch1/1 -> Switch/3
  Minus2/1 -> Switch1/1
  Relational Operator1/1 -> Switch1/2
  Gain/1 -> Relational Operator1/2
  Minus1/1 -> Relational Operator1/1
  Add/1 -> Switch/1
  Relational Operator/1 -> Switch/2
  Minus/1 -> Relational Operator/1
  Step/1 -> Relational Operator/2, Add/1, Gain/1, Minus2/2
  ResDelay/1 -> Minus/2, Add/2, Minus2/1, Minus1/2
  Ref/1 -> Minus/1, Minus1/1, Switch1/3

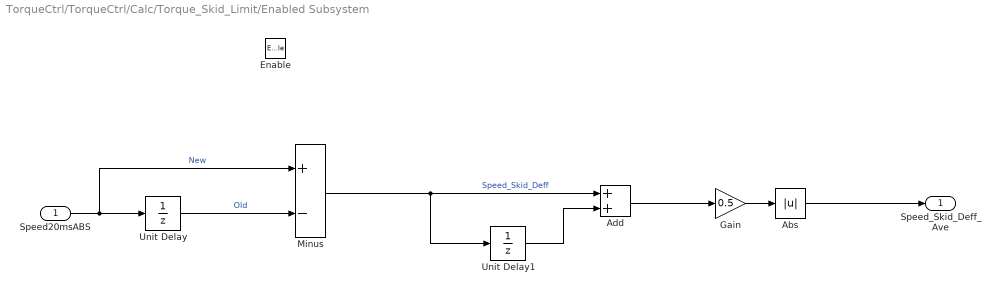
== system TorqueCtrl/TorqueCtrl/Calc/Torque_Skid_Limit/Enabled Subsystem ==
  Speed20msABS : Inport
  Enable : EnablePort
  Abs : Abs  SaturateOnIntegerOverflow=off
  Add : Sum
  Gain : Gain  Gain=0.5  ParamDataTypeStr=single  OutDataTypeStr=single
  Minus : Sum  Inputs=+-
  Unit Delay : UnitDelay  SampleTime=-1  HasFrameUpgradeWarning=on
  Unit Delay1 : UnitDelay  SampleTime=-1  HasFrameUpgradeWarning=on
  Speed_Skid_Deff_Ave : Outport
  wires:
  Speed20msABS/1 -> Minus/1, Unit Delay/1  "New"
  Unit Delay/1 -> Minus/2  "Old"
  Minus/1 -> Unit Delay1/1, Add/1  "Speed_Skid_Deff"
  Add/1 -> Gain/1
  Unit Delay1/1 -> Add/2
  Gain/1 -> Abs/1
  Abs/1 -> Speed_Skid_Deff_Ave/1

== stateflow chart TorqueCtrl/Calc/Torque_Skid_Limit/Chart1 ==
  (default) -> (junction 130)
  (junction 130) -> (junction 132) [order 1] : [Speed20msABS > 200]
  (junction 130) -> (junction 139) [order 2] : {
      | Out = TorqueCmdLimit;
      | SkidExitCnt = 0;
      | SpeedSkidFlag =0;
      | }
  (junction 132) -> (junction 135)
  (junction 135) -> (junction 3)
  (junction 3) -> (junction 5) [order 1] : [Speed_Skid_Deff_Ave>100]
  (junction 3) -> (junction 12) [order 2]
  (junction 5) -> (junction 7) : {
      | Out = TorqueCmdLimit*100/Speed_Skid_Deff_Ave;
      | SpeedSkidFlag = 1;
      | SkidExitCnt = 0;
      | }
  (junction 7) -> (junction 98)
  (junction 12) -> (junction 57) [order 1] : [Speed_Skid_Deff_Ave < 50]
  (junction 12) -> (junction 77) [order 2]
  (junction 57) -> (junction 59) : {
      | Out = TorqueCmdLimit;
      | }
  (junction 59) -> (junction 61) [order 1] : [SpeedSkidFlag ==1]{SkidExitCnt = SkidExitCnt +1}
  (junction 61) -> (junction 64) [order 1] : [SkidExitCnt>=200]{SpeedSkidFlag = 0;SkidExitCnt=0}
  (junction 61) -> (junction 64) [order 2]
  (junction 59) -> (junction 61) [order 2]
  (junction 64) -> (junction 67)
  (junction 77) -> (junction 69) [order 1] : {SkidExitCnt=0}
  (junction 69) -> (junction 71) [order 1] : [SpeedSkidFlag==0]
  (junction 77) -> (junction 95) [order 2]
  (junction 69) -> (junction 79) [order 2]
  (junction 71) -> (junction 73) : {
      | Out = TorqueCmdLimit;
      | SkidExitCnt = 0;
      |
      | }
  (junction 73) -> (junction 87)
  (junction 79) -> (junction 81) [order 1] : [abs(OutDelay)>abs(TorqueCmdLimit)]{Out = TorqueCmdLimit;SkidExitCnt = 0}
  (junction 79) -> (junction 81) [order 2]
  (junction 81) -> (junction 85)
  (junction 87) -> (junction 85)
  (junction 85) -> (junction 90)
  (junction 90) -> (junction 95)
  (junction 67) -> (junction 90)
  (junction 98) -> (junction 67)
  (junction 95) -> (junction 102)
  (junction 102) -> (junction 139)
  (junction 139) -> (junction 137)
  data: Speed20msABS input; TorqueCmdLimit input; Speed_Skid_Deff_Ave input; Out output single =0; OutDelay input; SkidExitCnt local uint8 =0; SpeedSkidFlag local uint8 =0

== stateflow chart TorqueCtrl/Calc/Torque_Skid_Limit/Chart ==
  (default) -> (junction 1) : {Cnt = Cnt + 1}
  (junction 1) -> (junction 3) [order 1] : [Cnt >= 5]
  (junction 1) -> (junction 8) [order 2] : {En = 0}
  (junction 3) -> (junction 6) : {Cnt = 0
      | En = 1}
  (junction 6) -> (junction 8)
  (junction 8) -> (junction 13)
  data: Cnt local uint8 =0; En output uint8 =0
